simulink model "vdp2d"  (Simulink 8.4)
settings: Solver=ode45  SolverMode=SingleTasking  StartTime=0.0  StopTime=100  RelTol=1e-3  AbsTol=1e-6
settings Model: Creator=The MathWorks Inc.  LastModifiedBy=gcampa  ExtModeTrigMode=oneshot  ExtModeArmWhenConnect=off
settings DataIOCC: ExternalInput=[]  InitialState=[]  LimitDataPoints=off  SaveOutput=off  SaveTime=off
settings OptimizationCC: BlockReduction=off  BooleanDataType=off  ExpressionDepthLimit=128  InitFltsAndDblsToZero=on
settings DebuggingCC: SaveWithParameterizedLinksMsg=none  SignalResolutionControl=TryResolveAllWithWarning  SolverPrmCheckMsg=none  MultiTaskDSMMsg=warning  MultiTaskCondExecSysMsg=none  IntegerOverflowMsg=none  FcnCallInpInsideContextMsg=EnableAllAsError  FrameProcessingCompatibilityMsg=error  StateNameClashWarn=none
settings HardwareCC: TargetUnknown=on
settings GRTTargetCC: TargetFcnLib=ansi_tfl_tmw.mat
settings ConfigComp: CovMetricSettings=dw  CovHtmlReporting=on  CovSaveCumulativeToWorkspaceVar=on  CovSaveSingleToWorkspaceVar=on  CovModelRefEnable=Off  CovExternalEMLEnable=off  CovSFcnEnable=off

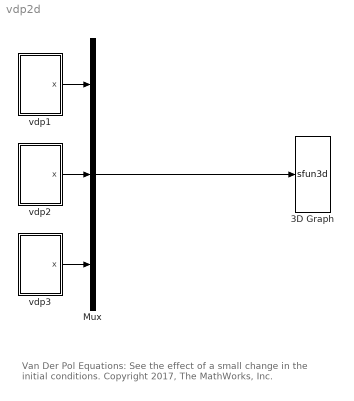
== system vdp2d ==
  note: Van Der Pol Equations:
      | See the effect of a small change in the initial conditions.
      | Copyright 2017, The MathWorks, Inc.
  3D Graph : S-Function  LoadFcn=if exist('sfun3d','file'), sfun3d([],[],[],'LoadBlock'); end  FunctionName=sfun3d  Parameters=ax,T,np,cp,gd,ls,mk,mx,hd,tb  EnableBusSupport=off  mask(3D Graph){np=3, ax=[-3 3 -6 6 0 1], mx=200, T=0.01, cp=[0 0 1], gd=on, hd=on, tb=off, ls=-, mk=none}
      mask prompts: np "Number of moving points (lines)"; ax "Range: [xmin xmax  ymin ymax zmin zmax]"; mx "Max number of points in each line"; T "Sampling Time"; cp "Camera position (use [0 0 1] for 2D XY view)"; gd "Grid (on|off)"; hd "HeadMarkers (on|off)"; tb "Toolbar (on|off)"; ls "LineStyle"; mk "LineMarker"
      mask help:
      | This block plots the position of several points in the XYZ space. The input contains the coordinates of all the points (x1,y1,z1,x2,y2,z2,...).
      | The number of moving points (lines), the XYZ ranges, sampling time, camera position, and grid (among other things) can be set as mask parameters.
      settings: CopyFcn=if exist('sfun3d','file'), sfun3d([],[],[],'CopyBlock'); end  DeleteFcn=if exist('sfun3d','file'), sfun3d([],[],[],'DeleteBlock'); end  NameChangeFcn=if exist('sfun3d','file'), sfun3d([],[],[],'NameChange'); end
      mask Help:
      | This block plots the position of several points in the XYZ space. The input contains the coordinates of all the points (x1,y1,z1,x2,y2,z2,...).
      | The number of moving points (lines), the XYZ ranges, sampling time, camera position, and grid (among other things) can be set as mask parameters.
      mask TypeOptions ls: - | -- | : | -. | none
      mask TypeOptions mk: none | . | + | o | * | x | square | diamond | v | ^ | > | < | pentagram | hexagram
      mask Display: plot([.05 .95 .95 .05 .05],[.45 .45 .95 .95 .45], 0.5+cos(0:0.1:2*pi)*0.3,0.7+sin(0:0.1:2*pi)*0.2)
  Mux : Mux  Inputs=[3 3 3]
  vdp1 : Subsystem  mask(Van Der Pol System){mu=1, x0=[1 0]}
      mask prompts: x0 "Initial Conditions [p0 v0]"
      mask help: Van Der Pol Oscillator System: xdotdot=mu*xdot*(1-x^2)-x
      mask Help: Van Der Pol Oscillator System: xdotdot=mu*xdot*(1-x^2)-x
  vdp2 : Subsystem  mask(Van Der Pol System){mu=1.5, x0=[1 0]}
      mask prompts: x0 "Initial Conditions [p0 v0]"
      mask help: Van Der Pol Oscillator System: xdotdot=mu*xdot*(1-x^2)-x
      mask Help: Van Der Pol Oscillator System: xdotdot=mu*xdot*(1-x^2)-x
  vdp3 : Subsystem  mask(Van Der Pol System){mu=2.5, x0=[1 0]}
      mask prompts: x0 "Initial Conditions [p0 v0]"
      mask help: Van Der Pol Oscillator System: xdotdot=mu*xdot*(1-x^2)-x
      mask Help: Van Der Pol Oscillator System: xdotdot=mu*xdot*(1-x^2)-x
  wires:
  vdp1/1(x) -> Mux/1
  vdp2/1(x) -> Mux/2
  vdp3/1(x) -> Mux/3
  Mux/1 -> 3D Graph/1

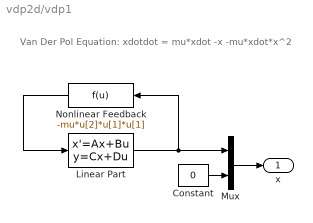
== system vdp2d/vdp1 ==
  note: Van Der Pol Equation: xdotdot = mu*xdot -x -mu*xdot*x^2
  Constant : Constant  Value=0
  Linear Part : StateSpace  A=[0 1; -1 mu]  B=[0 1]'  C=eye(2)  D=[0 0]'  X0=x0
  Mux : Mux  Inputs=[2 1]
  Nonlinear Feedback : Fcn  Expr=-mu*u[2]*u[1]*u[1]
  x : Outport
  wires:
  Linear Part/1 -> Mux/1, Nonlinear Feedback/1
  Nonlinear Feedback/1 -> Linear Part/1
  Constant/1 -> Mux/2
  Mux/1 -> x/1

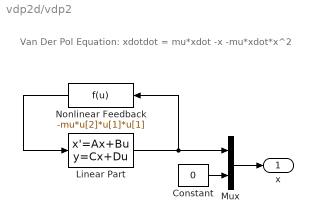
== system vdp2d/vdp2 ==
  note: Van Der Pol Equation: xdotdot = mu*xdot -x -mu*xdot*x^2
  Constant : Constant  Value=0
  Linear Part : StateSpace  A=[0 1; -1 mu]  B=[0 1]'  C=eye(2)  D=[0 0]'  X0=x0
  Mux : Mux  Inputs=[2 1]
  Nonlinear Feedback : Fcn  Expr=-mu*u[2]*u[1]*u[1]
  x : Outport
  wires:
  Mux/1 -> x/1
  Constant/1 -> Mux/2
  Nonlinear Feedback/1 -> Linear Part/1
  Linear Part/1 -> Nonlinear Feedback/1, Mux/1

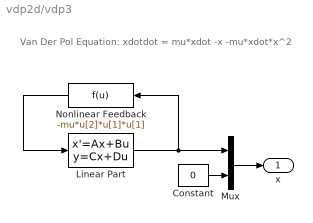
== system vdp2d/vdp3 ==
  note: Van Der Pol Equation: xdotdot = mu*xdot -x -mu*xdot*x^2
  Constant : Constant  Value=0
  Linear Part : StateSpace  A=[0 1; -1 mu]  B=[0 1]'  C=eye(2)  D=[0 0]'  X0=x0
  Mux : Mux  Inputs=[2 1]
  Nonlinear Feedback : Fcn  Expr=-mu*u[2]*u[1]*u[1]
  x : Outport
  wires:
  Linear Part/1 -> Mux/1, Nonlinear Feedback/1
  Nonlinear Feedback/1 -> Linear Part/1
  Constant/1 -> Mux/2
  Mux/1 -> x/1
